simulink model "charge_circuit_12v"  (R2021b)
settings: Solver=VariableStepAuto  StartTime=0.0  StopTime=560  RelTol=1e-3
undefined symbols (not defined in the file): Ion, Lithium
libraries: spsBatteryLib x3, spsDCVoltageSourceLib x1, spsIGBTDiodeLib x1, spsVoltageMeasurementLib x1, spspowerguiLib x1
settings Model: Creator=AishwaryaSalunke  LastModifiedBy=Admin
settings SolverCC: ZeroCrossAlgorithm=Adaptive  AlgebraicLoopSolver=TrustRegion
settings DataIOCC: ReturnWorkspaceOutputs=off
settings DebuggingCC: MaxConsecutiveZCsMsg=none  SFMachineParentedDataDiag=warning  ArithmeticOperatorsInVariantConditions=warning
settings SFSimCC: SimUseLocalCustomCode=off  CustomCodeUndefinedFunction=UseInterfaceOnly
settings RTWCC: RTWUseLocalCustomCode=off

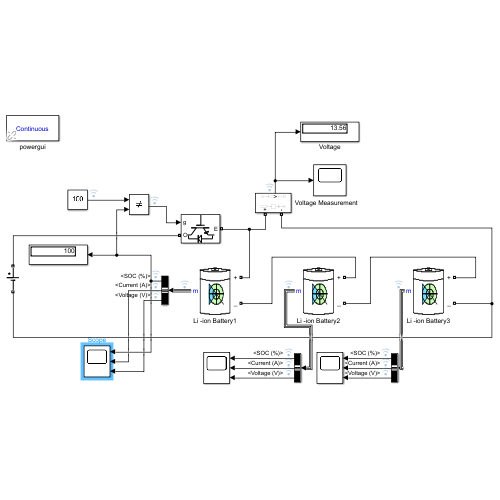
[thumbnail: Simulink's stored preview of the top-level diagram]
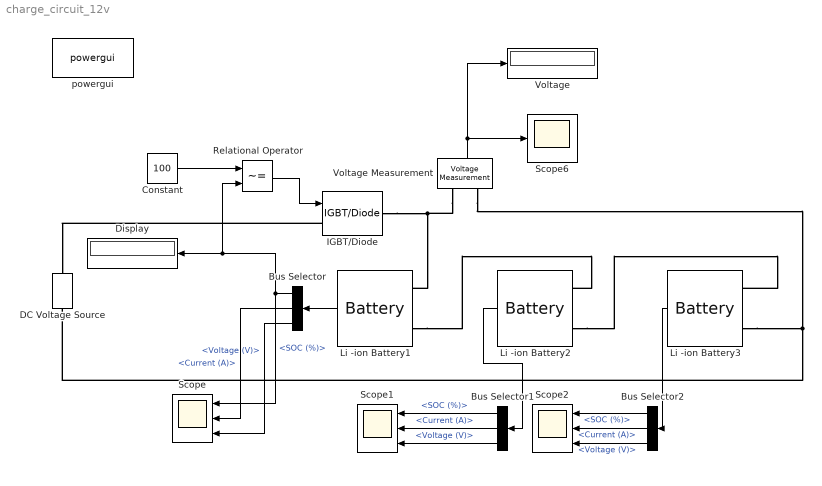
== system charge_circuit_12v ==
  Bus Selector : BusSelector  OutputSignals=SOC (%),Current (A),Voltage (V)
  Bus Selector1 : BusSelector  OutputSignals=SOC (%),Current (A),Voltage (V)
  Bus Selector2 : BusSelector  OutputSignals=SOC (%),Current (A),Voltage (V)
  Constant : Constant  Value=100
  DC Voltage Source : spsDCVoltageSourceLib/DC Voltage Source  Amplitude=14  Measurements=None
  Display : Display
  IGBT/Diode : spsIGBTDiodeLib/IGBT//Diode  Ron=1e-3  Rs=1e5  Cs=inf  Measurements=off
  Li -ion Battery1 : spsBatteryLib/Battery  BatType=Lithium-Ion  ShowTempParam=off  ThermalPreset=no  ShowAgeParam=off  NomV=3.7  NomQ=2.6  SOC=10  Batt_Tr=30  PresetModel=on  MaxQ=2.6  MinV=2.775  FullV=4.3068  Dis_rate=1.1304  R=0.014231  Normal_OP=2.3513  expZone="[3.9974     0.12774]"  current=[6.5 13 32.5]  Units=Time  Tci=20  NomT=20  T2=-30  MaxQ2=4.8  FullV2=7.1  Normal_OP2=5.655  expZone2="[6.58           1]"  Rca=0.6  ti=2000  Dp=0  Neq0=0  Tsim=1e6  Ta1=25  Qeol=5.4*0.9  Reol=0.013333*1.2  Char_age=[2.3478, 3]  Dis_age=[2.3478, 10]  N1=1500  N2=10500  N3=1000  N4=1400  Ta2=45  N5=950
  Li -ion Battery2 : spsBatteryLib/Battery  BatType=Lithium-Ion  ShowTempParam=off  ThermalPreset=no  ShowAgeParam=off  NomV=3.7  NomQ=2.6  SOC=10  Batt_Tr=30  PresetModel=on  MaxQ=2.6  MinV=2.775  FullV=4.3068  Dis_rate=1.1304  R=0.014231  Normal_OP=2.3513  expZone="[3.9974     0.12774]"  current=[6.5 13 32.5]  Units=Time  Tci=20  NomT=20  T2=-30  MaxQ2=4.8  FullV2=7.1  Normal_OP2=5.655  expZone2="[6.58           1]"  Rca=0.6  ti=2000  Dp=0  Neq0=0  Tsim=1e6  Ta1=25  Qeol=5.4*0.9  Reol=0.013333*1.2  Char_age=[2.3478, 3]  Dis_age=[2.3478, 10]  N1=1500  N2=10500  N3=1000  N4=1400  Ta2=45  N5=950
  Li -ion Battery3 : spsBatteryLib/Battery  BatType=Lithium-Ion  ShowTempParam=off  ThermalPreset=no  ShowAgeParam=off  NomV=3.7  NomQ=2.6  SOC=10  Batt_Tr=30  PresetModel=on  MaxQ=2.6  MinV=2.775  FullV=4.3068  Dis_rate=1.1304  R=0.014231  Normal_OP=2.3513  expZone="[3.9974     0.12774]"  current=[6.5 13 32.5]  Units=Time  Tci=20  NomT=20  T2=-30  MaxQ2=4.8  FullV2=7.1  Normal_OP2=5.655  expZone2="[6.58           1]"  Rca=0.6  ti=2000  Dp=0  Neq0=0  Tsim=1e6  Ta1=25  Qeol=5.4*0.9  Reol=0.013333*1.2  Char_age=[2.3478, 3]  Dis_age=[2.3478, 10]  N1=1500  N2=10500  N3=1000  N4=1400  Ta2=45  N5=950
  Relational Operator : RelationalOperator  Operator=~=  OutDataTypeStr=boolean  RndMeth=Simplest
  Scope : Scope  NumInputPorts=3
  Scope1 : Scope  NumInputPorts=3
  Scope2 : Scope  NumInputPorts=3
  Scope6 : Scope
  Voltage : Display
  Voltage Measurement : spsVoltageMeasurementLib/Voltage Measurement  PhasorSimulation=off  OutputType=Complex  PSBequivalent=0
  powergui : spspowerguiLib/powergui  Priority=1  SimulationMode=Continuous  SampleTime=50e-6  frequency=60  Iterations=50  frequencyindice=0  Pbase=100e6  ErrMax=1e-4  UnitsV=kV  UnitsW=MW  buscounter=0  FunctionMessages=off  echomessages=off  EnableUseOfTLC=off  CurrentSourceSwitches=off  DisableSnubberDevices=off  DisableRonSwitches=off  DisableVfSwitches=off  DisplayEquations=off  AutomaticDiscreteSolvers=off  SolverType=Tustin/Backward Euler (TBE)  Interpol=off  ExternalGateDelay=off  methode=off  Ts=100  x0status=blocks  SPID=on  SwTol=0  HookPort=off  NonlinearTolerance=1e-4  nMaxIteration=100  ContinueOnMaxIteration=off  RestoreLinks=warning  ResistiveCurrentMeasurement=off  Frange=[0:2:500]  Ylog=off  Xlog=on  ShowGrid=off  save=off  variable=ZData  structure=0  ZoomFFT=off  StartTime=0.0  cycles=1  DisplayStyle=1  fundamental=60  FreqAxis=off  MaxFrequency=1000  frequencyindicesteady=1  RmsSteady=1  display=off
  wires:
  Bus Selector/1 -> Display/1, Relational Operator/2, Scope/1  "<SOC (%)>"
  Bus Selector/2 -> Scope/2  "<Current (A)>"
  Bus Selector/3 -> Scope/3  "<Voltage (V)>"
  Li -ion Battery1/1 -> Bus Selector/1
  Voltage Measurement/1 -> Voltage/1, Scope6/1
  Relational Operator/1 -> IGBT/Diode/1
  Constant/1 -> Relational Operator/1
  Bus Selector2/1 -> Scope2/1  "<SOC (%)>"
  Bus Selector2/2 -> Scope2/2  "<Current (A)>"
  Bus Selector2/3 -> Scope2/3  "<Voltage (V)>"
  Li -ion Battery3/1 -> Bus Selector2/1
  Li -ion Battery2/1 -> Bus Selector1/1
  Bus Selector1/1 -> Scope1/1  "<SOC (%)>"
  Bus Selector1/2 -> Scope1/2  "<Current (A)>"
  Bus Selector1/3 -> Scope1/3  "<Voltage (V)>"
  connections:
  Li -ion Battery1/LConn2 -- Li -ion Battery2/LConn1
  Li -ion Battery2/LConn2 -- Li -ion Battery3/LConn1
  IGBT/Diode/RConn1 -- Li -ion Battery1/LConn1 -- Voltage Measurement/LConn1
  IGBT/Diode/LConn1 -- DC Voltage Source/RConn1
  Li -ion Battery3/LConn2 -- DC Voltage Source/LConn1 -- Voltage Measurement/LConn2
